simulink model "GainScheduled_PID_Controller"  (R2020a)
settings: Solver=FixedStepDiscrete  StartTime=0.0  StopTime=SimEndTime  FixedStep=TimeStep  RelTol=1e-3
undefined symbols (not defined in the file): ctrl_start_time, deadzone_comp_flag, deadzone_comp_val, I_gain_init, I_gain_table, Iout_op, P_gain_init, P_gain_table, TimeStep
libraries: simulink x1
settings Model: DataDictionary=system_data.sldd  Creator=tshintai  LastModifiedBy=tshintai
settings DataIOCC: SaveOutput=off  SaveTime=off

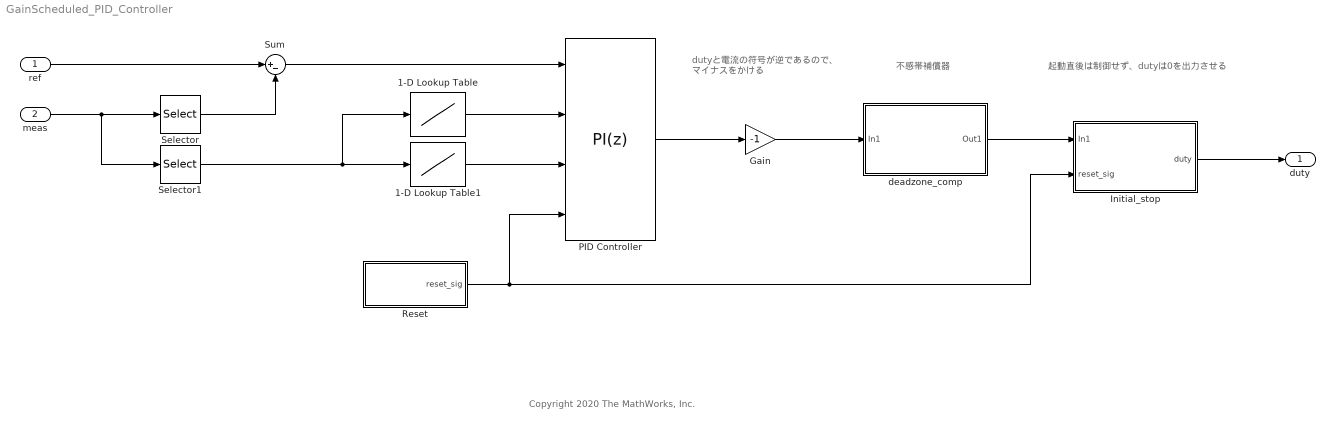
== system GainScheduled_PID_Controller ==
  note: Copyright 2020 The MathWorks, Inc.
  note: dutyと電流の符号が逆であるので、
      | マイナスをかける
  note: 起動直後は制御せず、dutyは0を出力させる
  note: 不感帯補償器
  ref : Inport  OutDataTypeStr=double  PortDimensions=1  SampleTime=[0.0001,0]
  meas : Inport  Port=2  OutDataTypeStr=double  PortDimensions=3  SampleTime=[0.0001,0]
  1-D Lookup Table : Lookup_n-D  NumberOfTableDimensions=1  BreakpointsForDimension1=Iout_op  Table=P_gain_table  ExtrapMethod=Clip  InternalRulePriority=Speed  RndMeth=Simplest  InputSameDT=on
  1-D Lookup Table1 : Lookup_n-D  NumberOfTableDimensions=1  BreakpointsForDimension1=Iout_op  Table=I_gain_table  ExtrapMethod=Clip  InternalRulePriority=Speed  RndMeth=Simplest  InputSameDT=on
  Gain : Gain  Gain=-1
  Initial_stop : Subsystem
  PID Controller : simulink/Continuous/PID Controller  Controller=PI  Form=Parallel  TimeDomain=Discrete-time  UseExternalTs=off  SampleTime=-1  IntegratorMethod=Forward Euler  FilterMethod=Forward Euler  ControllerParametersSource=external  P=P_gain_init  I=I_gain_init  D=0  UseFilter=on  N=100  TunerSelectOption=Transfer Function Based (PID Tuner App)  InitialConditionSource=internal  InitialConditionForIntegrator=0  InitialConditionForFilter=0  DifferentiatorICPrevScaledInput=0  ExternalReset=level  TrackingMode=off  Kt=1  LimitOutput=on  UpperSaturationLimit=0.7  LowerSaturationLimit=-0.7  LinearizeAsGain=on  AntiWindupMode=clamping  Kb=1  POutMin=[]  POutMax=[]  IOutMin=[]  IOutMax=[]  DOutMin=[]  DOutMax=[]  NOutMin=[]  NOutMax=[]  SumOutMin=[]  SumOutMax=[]  SaturationOutMin=[]  SaturationOutMax=[]  PParamMin=[]  PParamMax=[]  IParamMin=[]  IParamMax=[]  DParamMin=[]  DParamMax=[]  NParamMin=[]  NParamMax=[]  KbParamMin=[]  KbParamMax=[]  KtParamMin=[]  KtParamMax=[]  KbOutMin=[]  KbOutMax=[]  KtOutMin=[]  KtOutMax=[]  IntegratorOutMin=[]  IntegratorOutMax=[]  FilterOutMin=[]  FilterOutMax=[]  SumI1OutMin=[]  SumI1OutMax=[]  SumI2OutMin=[]  SumI2OutMax=[]  SumI3OutMin=[]  SumI3OutMax=[]  SumI4OutMin=[]  SumI4OutMax=[]  SumDOutMin=[]  SumDOutMax=[]  DifferentiatorOutMin=[]  DifferentiatorOutMax=[]  FilterDiffOutCoefMin=[]  FilterDiffOutCoefMax=[]  ReciprocalOutMin=[]  ReciprocalOutMax=[]  SumDenOutMin=[]  SumDenOutMax=[]  SumNumOutMin=[]  SumNumOutMax=[]  DivideOutMin=[]  DivideOutMax=[]  UdiffTsProdOutMin=[]  UdiffTsProdOutMax=[]  NTsProdOutMin=[]  NTsProdOutMax=[]  UintegralTsProdOutMin=[]  UintegralTsProdOutMax=[]  UngainTsProdOutMin=[]  UngainTsProdOutMax=[]  IntegratorContinuousStateAttributes=''  IntegratorStateMustResolveToSignalObject=off  IntegratorRTWStateStorageClass=Auto  FilterContinuousStateAttributes=''  FilterStateMustResolveToSignalObject=off  FilterRTWStateStorageClass=Auto  ParallelPVariant=ExternalParameters  IdealPVariant=Disabled  IVariant=ExternalParameters  DVariant=Disabled  IntegratorVariant=Discrete  SatVariant=Enabled  AWVariant=DiscClampingParallel  PCopyVariant=Disabled  TRVariant=Disabled  FdbkBlocksVariant=Forward  IdealPFdbkVariant=Disabled  SatFdbkVariant=Disabled  DerivativeFilterVariant=Disabled  NVariant=Disabled  NCopyVariant=Disabled_SignalSpec  FilterICVariant=Disabled  IntegratorICVariant=InternalICs  ExternalResetVariant=ExternalReset  TRSumVariant=Passthrough  SumFdbkVariant=Disabled  SumVariant=Sum_PI  TsampFilterVariant=InternalTs  TsampNgainVariant=Passthrough  TsampIntegralVariant=Passthrough
  Reset : Subsystem
  Selector : Selector  InputPortWidth=3  IndexOptions=Index vector (dialog)  Indices=[2]  OutputSizes=1
  Selector1 : Selector  InputPortWidth=3  IndexOptions=Index vector (dialog)  Indices=[3]  OutputSizes=1
  Sum : Sum  Inputs=|+-
  deadzone_comp : Subsystem
  duty : Outport  OutDataTypeStr=double  PortDimensions=1  SampleTime=[0.0001,0]
  wires:
  ref/1 -> Sum/1
  meas/1 -> Selector/1, Selector1/1
  Selector/1 -> Sum/2
  Sum/1 -> PID Controller/1
  PID Controller/1 -> Gain/1
  Gain/1 -> deadzone_comp/1(In1)
  Reset/1(reset_sig) -> Initial_stop/2(reset_sig), PID Controller/4
  Initial_stop/1(duty) -> duty/1
  deadzone_comp/1(Out1) -> Initial_stop/1(In1)
  1-D Lookup Table/1 -> PID Controller/2
  1-D Lookup Table1/1 -> PID Controller/3
  Selector1/1 -> 1-D Lookup Table/1, 1-D Lookup Table1/1

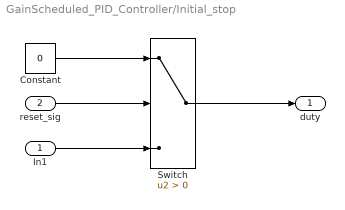
== system GainScheduled_PID_Controller/Initial_stop ==
  In1 : Inport
  reset_sig : Inport  Port=2
  Constant : Constant  Value=0
  Switch : Switch  Criteria=u2 > Threshold
  duty : Outport
  wires:
  reset_sig/1 -> Switch/2
  Switch/1 -> duty/1
  Constant/1 -> Switch/1
  In1/1 -> Switch/3

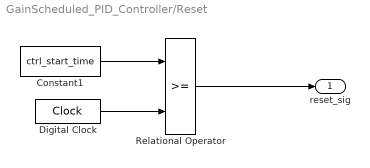
== system GainScheduled_PID_Controller/Reset ==
  Constant1 : Constant  Value=ctrl_start_time
  Digital Clock : DigitalClock  SampleTime=TimeStep
  Relational Operator : RelationalOperator  OutDataTypeStr=boolean  RndMeth=Simplest
  reset_sig : Outport
  wires:
  Relational Operator/1 -> reset_sig/1
  Digital Clock/1 -> Relational Operator/2
  Constant1/1 -> Relational Operator/1

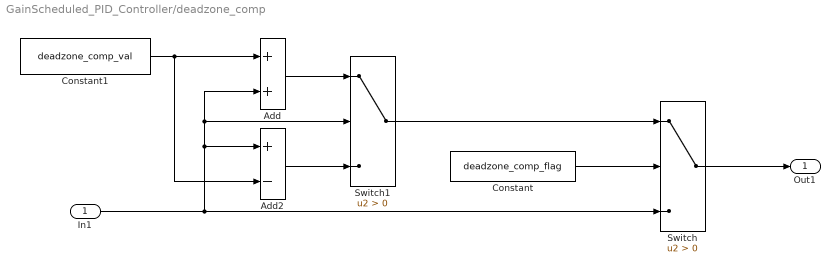
== system GainScheduled_PID_Controller/deadzone_comp ==
  In1 : Inport
  Add : Sum
  Add2 : Sum  Inputs=+-
  Constant : Constant  Value=deadzone_comp_flag
  Constant1 : Constant  Value=deadzone_comp_val
  Switch : Switch  Criteria=u2 > Threshold
  Switch1 : Switch  Criteria=u2 > Threshold
  Out1 : Outport
  wires:
  Switch/1 -> Out1/1
  In1/1 -> Add/2, Switch1/2, Add2/1, Switch/3
  Constant/1 -> Switch/2
  Add/1 -> Switch1/1
  Constant1/1 -> Add2/2, Add/1
  Add2/1 -> Switch1/3
  Switch1/1 -> Switch/1
